simulink model "lrlowpass_6"  (R2016b)
settings: Solver=ode15s  StartTime=0.0  StopTime=50  RelTol=1e-3
values from neighbouring files (symbols this model uses):
  CH = 400    [rlcsolver_total.m]
  Ci = .0047    (= 0.0047)    [rlcsolver_total.m]
  CLw = 400    [rlcsolver_total.m]
  CM = 400    [rlcsolver_total.m]
  freq = 61    [rlcsolver_total.m]
  L1 = .02    (= 0.02)    [rlcsolver_total.m]
  n1 = 0.8/24    (= 0.0333333333333)    [rlcsolver_total.m]
  n2 = 0.45/24    (= 0.01875)    [rlcsolver_total.m]
  n3 = 0.25/24    (= 0.0104166666667)    [rlcsolver_total.m]
  PerT = 0.025    [rlcsolver_total.m]
  PerV = 12    [rlcsolver_total.m]
  R1 = .00192    (= 0.00192)    [rlcsolver_total.m]
  RH = 2.2e-6    (= 2.2e-06)    [rlcsolver_total.m]
  Ri = 1e-2    (= 0.01)    [rlcsolver_total.m]
  RLw = 6.94e-7    (= 6.94e-07)    [rlcsolver_total.m]
  RM = 1.24e-6    (= 1.24e-06)    [rlcsolver_total.m]
settings Model: Creator=Brian  LastModifiedBy=Brian

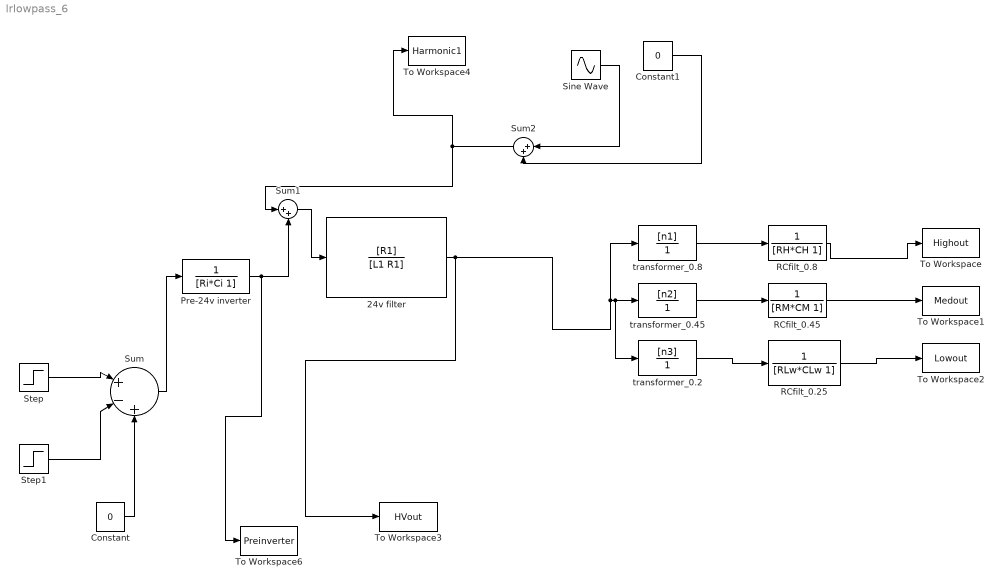
== system lrlowpass_6 ==
  24v filter : TransferFcn  Numerator=[R1]  Denominator=[L1 R1]
  Constant : Constant  Value=0
  Constant1 : Constant  Value=0
  Pre-24v inverter : TransferFcn  Denominator=[Ri*Ci 1]
  RCfilt_0.25 : TransferFcn  Denominator=[RLw*CLw 1]
  RCfilt_0.45 : TransferFcn  Denominator=[RM*CM 1]
  RCfilt_0.8 : TransferFcn  Denominator=[RH*CH 1]
  Sine Wave : Sin  Amplitude=.2  Frequency=6.28*freq  SampleTime=0
  Step : Step  Time=0  After=PerV  SampleTime=0
  Step1 : Step  Time=PerT  After=PerV  SampleTime=0
  Sum : Sum  Inputs=|+-+
  Sum1 : Sum  Inputs=|++
  Sum2 : Sum  Inputs=|++
  To Workspace : ToWorkspace  VariableName=Highout  SaveFormat=Timeseries  SampleTime=-1
  To Workspace1 : ToWorkspace  VariableName=Medout  SaveFormat=Timeseries  SampleTime=-1
  To Workspace2 : ToWorkspace  VariableName=Lowout  SaveFormat=Timeseries  SampleTime=-1
  To Workspace3 : ToWorkspace  VariableName=HVout  SaveFormat=Timeseries  SampleTime=-1
  To Workspace4 : ToWorkspace  VariableName=Harmonic1  SaveFormat=Timeseries  SampleTime=-1
  To Workspace6 : ToWorkspace  VariableName=Preinverter  SaveFormat=Timeseries  SampleTime=-1
  transformer_0.2 : TransferFcn  Numerator=[n3]  Denominator=[1]
  transformer_0.45 : TransferFcn  Numerator=[n2]  Denominator=[1]
  transformer_0.8 : TransferFcn  Numerator=[n1]  Denominator=[1]
  wires:
  24v filter/1 -> To Workspace3/1, transformer_0.8/1, transformer_0.2/1, transformer_0.45/1
  Step/1 -> Sum/1
  Step1/1 -> Sum/2
  Constant/1 -> Sum/3
  transformer_0.2/1 -> RCfilt_0.25/1
  transformer_0.45/1 -> RCfilt_0.45/1
  transformer_0.8/1 -> RCfilt_0.8/1
  RCfilt_0.8/1 -> To Workspace/1
  RCfilt_0.45/1 -> To Workspace1/1
  RCfilt_0.25/1 -> To Workspace2/1
  Sum2/1 -> To Workspace4/1, Sum1/1
  Sine Wave/1 -> Sum2/1
  Constant1/1 -> Sum2/2
  Sum1/1 -> 24v filter/1
  Sum/1 -> Pre-24v inverter/1
  Pre-24v inverter/1 -> To Workspace6/1, Sum1/2
